simulink model "test_rx_bf"  (R2020a)
settings: Solver=VariableStepAuto  StartTime=0.0  StopTime=30  RelTol=1e-3
undefined symbols (not defined in the file or in its folder): comm, constellation, frame, physconst, SDR, system
libraries: dspstat3 x4, commsync2 x3, dspsrcs4 x2, commsink2 x2, commdigbbndpm3 x2, commfilt2 x2, commsequence2 x2, phasedtxrxlib x2, commutil2 x2, commchan3 x1, commrflib2 x1, phasedbflib x1
settings Model: Creator=jose_  LastModifiedBy=jose_
settings DataIOCC: SignalLogging=off

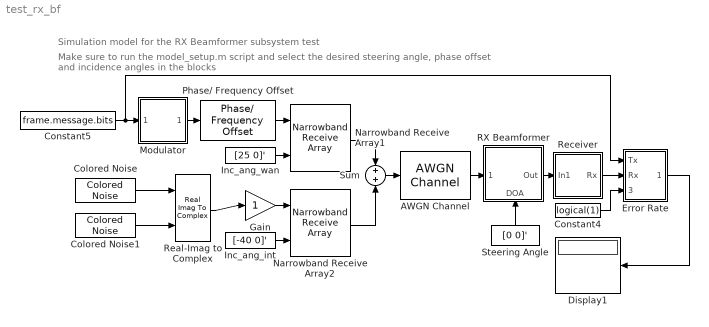
== system test_rx_bf ==
  note: Make sure to run the model_setup.m script and select the desired steering angle, phase offset and incidence angles in the blocks
  note: Simulation model for the RX Beamformer subsystem test
  AWGN Channel : commchan3/AWGN Channel  InputProcessing=Columns as channels (frame based)  seed=67  noiseMode="Signal to noise ratio  (SNR)"  EbNodB=20  EsNodB=10  SNRdB=10  bitsPerSym=2  Ps=1  Tsym=0.01/10000  variance=1
  Colored Noise : dspsrcs4/Colored Noise  Color=white  InverseFrequencyPower=1  BoundedOutput=on  NumChannels=1  OutputDataType=double  SamplesPerFrame=10000  SampleTime=1/SDR.samplerate  RandomStream=mt19937ar with seed  Seed=67  SimulateUsing=Code generation
      settings: SourceProductBaseCode=DS
  Colored Noise1 : dspsrcs4/Colored Noise  Color=white  InverseFrequencyPower=1  BoundedOutput=on  NumChannels=1  OutputDataType=double  SamplesPerFrame=10000  SampleTime=1/SDR.samplerate  RandomStream=mt19937ar with seed  Seed=32  SimulateUsing=Code generation
      settings: SourceProductBaseCode=DS
  Constant4 : Constant  Value=logical(1)
  Constant5 : Constant  Value=frame.message.bits  SampleTime=system.step
  Display1 : Display
  Error Rate : Subsystem
  Gain : Gain
  Inc_ang_int : Constant  Value=[-40 0]'
  Inc_ang_wan : Constant  Value=[25 0]'
  Modulator : Subsystem
      mask Display: image('$imagefile'); % Use "Edit Image" on toolstrip to change.
  Narrowband Receive Array1 : phasedtxrxlib/Narrowband Receive Array  PropagationSpeed=physconst( 'LightSpeed' )  OperatingFrequency=system.freq  Wavefront=Plane  SensorGainMeasure=dBi  Polarization=None  WeightsInputPort=off  SimulateUsing=Code generation  Sensor=AntennaArray
      settings: SourceProductBaseCode=AR
  Narrowband Receive Array2 : phasedtxrxlib/Narrowband Receive Array  PropagationSpeed=physconst( 'LightSpeed' )  OperatingFrequency=system.freq  Wavefront=Plane  SensorGainMeasure=dBi  Polarization=None  WeightsInputPort=off  SimulateUsing=Code generation  Sensor=AntennaArray
      settings: SourceProductBaseCode=AR
  Phase/ Frequency Offset : commrflib2/Phase// Frequency Offset  phaseOffset=20  freqPort=off  freqOffset=0
  RX Beamformer : Subsystem
      settings: PortSchema="{\"entries\":[{\"content\":{\"sides\":[{\"content\":{\"connectorIds\":[\"In1\"]},\"type\":\"ConnectorPlacement.EquallySpacedRectSide\",\"uuid\":\"da6b99b9-07c1-40ec-94f6-5f8421c86696\"},{\"content\":{\"connectorIds\":[\"Out1\"],\"side\":\"RIGHT\"},\"type\":\"ConnectorPlacement.EquallySpacedRectSide\",\"uuid\":\"d1696111-4bb2-4715-9875-a9a0a5fdf0a8\"},{\"content\":{\"connectorIds\":[],\"side\":\"TOP\"},\"type\":\"ConnectorPlacement.EquallySpacedRectSide\",\"uuid\":\"2098a05d-1eb1-4caf-b28b-c43268db6279\"},{\"content\":{\"connectorIds\":[\"In2\"],\"side\":\"BOTTOM\"},\"type\":\"ConnectorPlacement.EquallySpacedRectSide\",\"uuid\":\"baaf1a26-1617-49ff-8044-4db1bbf8bae7\"}]},\"type\":\"ConnectorPlacement.EquallySpacedConnector\",\"uuid\":\"7953a551-d915-4cd7-8910-f2df4fb3e1ef\"}],\"packageUris\":[\"http://schema.mathworks.com/mf0/Connector/19700101\"],\"version\":\"1.0\"}"
      mask Display: image('$imagefile'); % Use "Edit Image" on toolstrip to change.
  Real-Imag to Complex : RealImagToComplex
  Receiver : Subsystem
      mask Display: image('$imagefile'); % Use "Edit Image" on toolstrip to change.
  Steering Angle : Constant  Value=[0 0]'  SampleTime=system.step
  Sum : Sum  Inputs=+|+
  wires:
  Colored Noise/1 -> Real-Imag to Complex/1
  Colored Noise1/1 -> Real-Imag to Complex/2
  RX Beamformer/1(Out) -> Receiver/1(In1)
  Inc_ang_wan/1 -> Narrowband Receive Array1/2
  Narrowband Receive Array2/1 -> Sum/2
  Narrowband Receive Array1/1 -> Sum/1
  Real-Imag to Complex/1 -> Gain/1
  Phase/ Frequency Offset/1 -> Narrowband Receive Array1/1
  Inc_ang_int/1 -> Narrowband Receive Array2/2
  Sum/1 -> AWGN Channel/1
  Steering Angle/1 -> RX Beamformer/2(DOA)
  Constant5/1 -> Error Rate/1(Tx), Modulator/1(Message)
  Constant4/1 -> Error Rate/3(Rst)
  Receiver/1(Rx) -> Error Rate/2(Rx)
  Error Rate/1(BER) -> Display1/1
  Gain/1 -> Narrowband Receive Array2/1
  Modulator/1(Out1) -> Phase/ Frequency Offset/1
  AWGN Channel/1 -> RX Beamformer/1(Array Input)

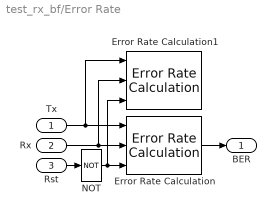
== system test_rx_bf/Error Rate ==
  Tx : Inport
  Rx : Inport  Port=2
  Rst : Inport  Port=3
  Error Rate Calculation : commsink2/Error Rate Calculation  N=0  st_delay=0  cp_mode=Entire frame  subframe=[]  PMode=Port  WsName=ErrorVec  RsMode2=on  stop=off  numErr=100  maxBits=1e6
  Error Rate Calculation1 : commsink2/Error Rate Calculation  N=0  st_delay=0  cp_mode=Entire frame  subframe=[]  PMode=Workspace  WsName=ErrorVec  RsMode2=on  stop=off  numErr=100  maxBits=1e6
  NOT : Logic  Operator=NOT  IconShape=distinctive  AllPortsSameDT=off  OutDataTypeStr=boolean
  BER : Outport
  wires:
  Tx/1 -> Error Rate Calculation1/1, Error Rate Calculation/1
  Rx/1 -> Error Rate Calculation1/2, Error Rate Calculation/2
  Error Rate Calculation/1 -> BER/1
  Rst/1 -> NOT/1
  NOT/1 -> Error Rate Calculation1/3, Error Rate Calculation/3

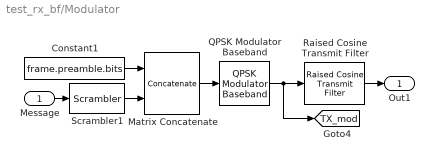
== system test_rx_bf/Modulator ==
  Message : Inport
  Constant1 : Constant  Value=frame.preamble.bits  SampleTime=system.step
  Matrix Concatenate : Concatenate  Mode=Multidimensional array
  QPSK Modulator Baseband : commdigbbndpm3/QPSK Modulator Baseband  InType=Bit  Enc=Gray  Ph=system.mod.PhaseOffset  outDtype=double  outWordLen=16  outUDDataType=sfix(16)  outFracLenMode=Best precision  outFracLen=15  outDataTypeStr=double  outLastDataTypeStr=double
  Raised Cosine Transmit Filter : commfilt2/Raised Cosine Transmit Filter  filtType=Square root  R=system.tx.rc.rolloff  filtSpan=system.tx.rc.span  N=system.tx.rc.interpolation  filterGain=sqrt(100)  InputProcessing=Columns as channels (frame based)  RateOptions=Enforce single-rate processing  framing=Mute  checkCoeff=off  variableName=rcTxFilt  checkGain=Normalized  sampMode=Mute  saveAsFlag=0  currentFiltSpan=system.tx.rc.span  D=(system.tx.rc.span)/2  launchFVT=on  roundingMode=Floor  overflowMode=off  coeffDataTypeStr=Inherit: Same word length as input  coeffMin=[]  coeffMax=[]  coeffLastDataTypeStr=Inherit: Same word length as input  outputDataTypeStr=Inherit: Same as accumulator  outputMin=[]  outputMax=[]  outputLastDataTypeStr=Inherit: Same as accumulator
  Scrambler1 : commsequence2/Scrambler  M=2  poly=[1 1 1 0 1]  iniStaSource=Dialog Parameter  ini_sta=[0 0 0 0]  resetViaPort=off
      settings: SourceProductBaseCode=CM
  Out1 : Outport
  tag scope: TX_mod=global
  wires:
  QPSK Modulator Baseband/1 -> [TX_mod], Raised Cosine Transmit Filter/1
  Matrix Concatenate/1 -> QPSK Modulator Baseband/1
  Raised Cosine Transmit Filter/1 -> Out1/1
  Constant1/1 -> Matrix Concatenate/1
  Message/1 -> Scrambler1/1
  Scrambler1/1 -> Matrix Concatenate/2

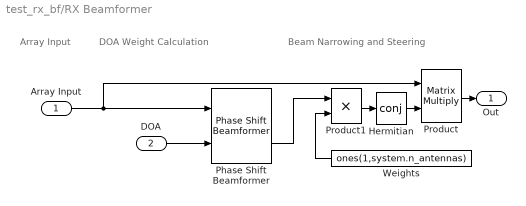
== system test_rx_bf/RX Beamformer ==
  note: Beam Narrowing and Steering
  note: DOA Weight Calculation
  note: Array Input
  Array Input : Inport
  DOA : Inport  Port=2
  Hermitian : Math  Operator=conj  SaturateOnIntegerOverflow=on
  Phase Shift Beamformer : phasedbflib/Phase Shift Beamformer  PropagationSpeed=physconst( 'LightSpeed' )  OperatingFrequency=system.freq  DirectionSource=Input port  Direction=[ 0; 0 ]  NumPhaseShifterBits=0  WeightsNormalization=Preserve power  WeightsOutputPort=on  SimulateUsing=Code generation  SensorArray=AntennaArray
      settings: SourceProductBaseCode=AR
  Product : Product  Multiplication=Matrix(*)
  Product1 : Product
  Weights : Constant  Value=ones(1,system.n_antennas)
  Out : Outport
  wires:
  Product1/1 -> Hermitian/1
  Hermitian/1 -> Product/2
  Product/1 -> Out/1
  Weights/1 -> Product1/2
  Phase Shift Beamformer/2 -> Product1/1
  Array Input/1 -> Product/1, Phase Shift Beamformer/1
  DOA/1 -> Phase Shift Beamformer/2

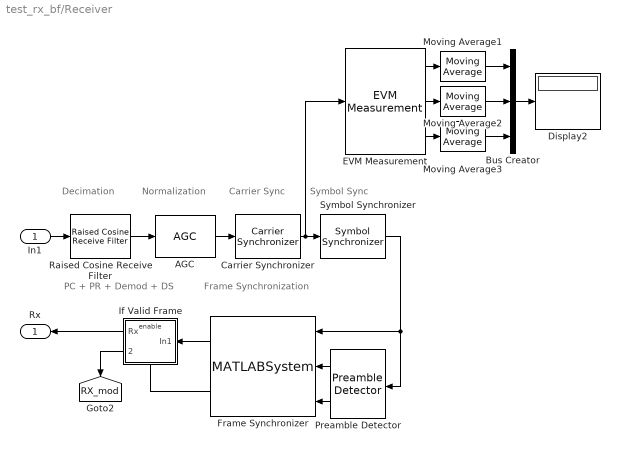
== system test_rx_bf/Receiver ==
  note: PC + PR + Demod + DS
  note: Frame Synchronization
  note: Symbol Sync
  note: Carrier Sync
  note: Normalization
  note: Decimation
  In1 : Inport
  AGC : commrfcorlib/AGC  LegacyMode=off  DetectorMethod=Rectifier  LoopMethod=Linear  UpdatePeriod=100  StepSize=0.1  AdaptationStepSize=system.rx.agc.step  DesiredOutputPower=system.rx.agc.output_power  AveragingLength=system.rx.agc.average_length  MaximumGain=30  MaxPowerGain=system.rx.agc.max_power  GainOutputPort=off  InputPowerOutputPort=off  SimulateUsing=Code generation
  Bus Creator : BusCreator  Inputs=3
  Carrier Synchronizer : commsync2/Carrier Synchronizer  Modulation=QPSK  ModulationPhaseOffset=Auto  CustomPhaseOffset=0  SamplesPerSymbol=system.rx.cs.sps  DampingFactor=system.rx.cs.damp  NormalizedLoopBandwidth=system.rx.cs.bandwidth  EstimatedPhaseErrorOutputPort=off  SimulateUsing=Code generation
  Display2 : Display
  EVM Measurement : commutil2/EVM Measurement  Normalization=Average reference signal power  AverageConstellationPower=1  PeakConstellationPower=1  ReferenceSignalSource=Estimated from reference constellation  ReferenceConstellation=constellation( comm.QPSKModulator )  MeasurementIntervalSource=Custom with periodic reset  MeasurementInterval=50  AveragingDimensions=1  MaximumEVMOutputPort=on  XPercentileEVMOutputPort=on  XPercentileValue=95  SymbolCountOutputPort=off  SimulateUsing=Code generation
      settings: SourceProductBaseCode=CM
  Frame Synchronizer : MATLABSystem  System=comm.internal.examples.FrameSynchronizer  Input=Symbol  OutputFrameLength=system.rx.fs.frame_length  PreambleLength=system.rx.fs.preamble_length  SimulateUsing=Code generation
      mask Type: comm.internal.examples.FrameSynchronizer
      mask Display:
      | disp(['Frame' char(10) 'Synchronizer']);
      | port_label('input',1,'u');
      | port_label('input',2,'idx');
      | port_label('input',3,'dtMt');
      | port_label('output',1,'Frame');
      | port_label('output',2,'Valid');
  If Valid Frame : Subsystem  TreatAsAtomicUnit=on
  Moving Average1 : dspstat3/Moving Average  Method=Sliding window  ForgettingFactorPort=off  SpecifyWindowLength=off  WindowLength=50  ForgettingFactor=0.9  SimulateUsing=Code generation
  Moving Average2 : dspstat3/Moving Average  Method=Sliding window  ForgettingFactorPort=off  SpecifyWindowLength=off  WindowLength=50  ForgettingFactor=0.9  SimulateUsing=Code generation
  Moving Average3 : dspstat3/Moving Average  Method=Sliding window  ForgettingFactorPort=off  SpecifyWindowLength=on  WindowLength=50  ForgettingFactor=0.9  SimulateUsing=Code generation
  Preamble Detector : commsync2/Preamble Detector  Input=Symbol  Preamble=system.rx.pd.preamble  Threshold=system.rx.pd.threshold  DetectionMetricOutput=on  Detections=All  SimulateUsing=Code generation
      settings: SourceProductBaseCode=CM
  Raised Cosine Receive Filter : commfilt2/Raised Cosine Receive Filter  filtType=Square root  R=system.rx.rc.rolloff  filtSpan=system.rx.rc.span  N=system.rx.rc.sps  downFactor=system.rx.rc.decimation  downOffset=0  filterGain=1  InputProcessing=Columns as channels (frame based)  RateOptions=Enforce single-rate processing  framing=Mute  checkCoeff=off  variableName=rcRxFilt  currentFiltSpan=system.rx.rc.span  D=(system.rx.rc.span)/2  inputOffset=0  sampMode=Mute  saveAsFlag=0  rateMode=Downsampling  checkGain=Normalized  launchFVT=on  roundingMode=Floor  overflowMode=off  coeffDataTypeStr=Inherit: Same word length as input  coeffMin=[]  coeffMax=[]  coeffLastDataTypeStr=Inherit: Same word length as input  accumDataTypeStr=Inherit: Same as product output  accumLastDataTypeStr=Inherit: Same as product output  outputDataTypeStr=Inherit: Same as accumulator  outputMin=[]  outputMax=[]  outputLastDataTypeStr=Inherit: Same as accumulator
  Symbol Synchronizer : commsync2/Symbol Synchronizer  Modulation=PAM/PSK/QAM  TimingErrorDetector=Zero-Crossing (decision-directed)  SamplesPerSymbol=system.rx.ss.sps  DampingFactor=system.rx.ss.damp  NormalizedLoopBandwidth=system.rx.ss.bandwidth  DetectorGain=system.rx.ss.gain  TimingErrorOutputPort=off  SimulateUsing=Code generation
      settings: SourceProductBaseCode=CM
  Rx : Outport
  tag scope: RX_mod=global
  wires:
  In1/1 -> Raised Cosine Receive Filter/1
  Raised Cosine Receive Filter/1 -> AGC/1
  Preamble Detector/1 -> Frame Synchronizer/2
  Frame Synchronizer/1 -> If Valid Frame/1(In1)
  If Valid Frame/1(Rx) -> Rx/1
  Frame Synchronizer/2 -> If Valid Frame/Enable
  AGC/1 -> Carrier Synchronizer/1
  Carrier Synchronizer/1 -> EVM Measurement/1, Symbol Synchronizer/1
  Preamble Detector/2 -> Frame Synchronizer/3
  Symbol Synchronizer/1 -> Frame Synchronizer/1, Preamble Detector/1
  If Valid Frame/2(pre-demod) -> [RX_mod]
  Moving Average2/1 -> Bus Creator/2
  Moving Average1/1 -> Bus Creator/1
  Moving Average3/1 -> Bus Creator/3
  EVM Measurement/3 -> Moving Average3/1
  EVM Measurement/1 -> Moving Average1/1
  EVM Measurement/2 -> Moving Average2/1
  Bus Creator/1 -> Display2/1

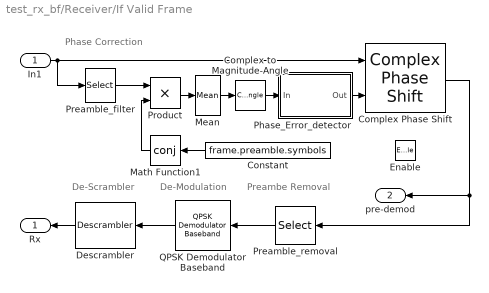
== system test_rx_bf/Receiver/If Valid Frame ==
  note: De-Scrambler
  note: De-Modulation
  note: Preambe Removal
  note: Phase Correction
  In1 : Inport
  Enable : EnablePort
  Complex Phase Shift : commutil2/Complex Phase Shift
      settings: SourceProductBaseCode=CM
  Complex to Magnitude-Angle : ComplexToMagnitudeAngle  Output=Angle
  Constant : Constant  Value=frame.preamble.symbols
  Descrambler : commsequence2/Descrambler  M=2  poly=[1 1 1 0 1]  iniStaSource=Dialog Parameter  ini_sta=[0 0 0 0]  resetViaPort=off
      settings: SourceProductBaseCode=CM
  Math Function1 : Math  Operator=conj  SignedPower=on  SaturateOnIntegerOverflow=on
  Mean : dspstat3/Mean  run=off  InputProcessing=Columns as channels (frame based)  reset_popup=None  directionMode=Each column  dimension=1  roiEnable=off  roiType=Rectangles  roiPortion=Entire ROI  roiOutput=Individual statistics for each ROI  roiFlag=off  roundingMode=Floor  overflowMode=off  outputDataTypeStr=Inherit: Same as accumulator  outputMin=[]  outputMax=[]  outputLastDataTypeStr=Inherit: Same as accumulator
  Phase_Error_detector : MATLAB Function  TreatAsAtomicUnit=on
  Preamble_filter : Selector  InputPortWidth=length(frame.symbols)  IndexOptions=Index vector (dialog)  Indices=1:length(frame.preamble.symbols)  OutputSizes=1
  Preamble_removal : Selector  InputPortWidth=length(frame.symbols)  IndexOptions=Index vector (dialog)  Indices=(length(frame.preamble.symbols)+1):length(frame.symbols)  OutputSizes=1
  Product : Product  RndMeth=Zero
  QPSK Demodulator Baseband : commdigbbndpm3/QPSK Demodulator Baseband  OutType=Bit  DecType=Hard decision  VarSource=Dialog  Variance=1  Dec=Gray  Ph=system.mod.PhaseOffset  outDtype1=Inherit via internal rule  outDtype2=Inherit via internal rule  derotateFactorWordLen=16  derotateFactorDataTypeStr=Inherit: Same word length as input  derotateFactorLastDataTypeStr=Inherit: Same word length as input
  Rx : Outport
  pre-demod : Outport  Port=2
  wires:
  Mean/1 -> Complex to Magnitude-Angle/1
  Product/1 -> Mean/1
  Complex to Magnitude-Angle/1 -> Phase_Error_detector/1(In)
  Preamble_filter/1 -> Product/1
  In1/1 -> Preamble_filter/1, Complex Phase Shift/1
  Constant/1 -> Math Function1/1
  Phase_Error_detector/1(Out) -> Complex Phase Shift/2
  Complex Phase Shift/1 -> Preamble_removal/1, pre-demod/1
  Math Function1/1 -> Product/2
  Preamble_removal/1 -> QPSK Demodulator Baseband/1
  QPSK Demodulator Baseband/1 -> Descrambler/1
  Descrambler/1 -> Rx/1

== matlab function test_rx_bf/Receiver/If Valid Frame/Phase_Error_detector ==
  data: In input; Out output
function Out = phasedecision(In)
% Map the estimated phase to one of -pi, -pi/2, 0, pi/2,  
%#codegen
Out = -round(In.*2./pi)./2.*pi;
% The above processing is equivalent to the following processing using
% if/else statements
%
% if In<pi/4 && In>-pi/4
%     Out = 0;
% elseif In>=pi/4 && In<pi*3/4
%     Out = pi/2;
% elseif In>=pi*3/4 || In<=-pi*3/4
%     Out = -pi;
% else
%     Out = -pi/2;
% end
